simulink model "Solar_Plant_Harness"  (R2025b)
settings: Solver=VariableStepAuto  StartTime=0.0  StopTime=5  RelTol=1e-3
PostLoadFcn:
  | SolarPlantParam;
values from neighbouring files (symbols this model uses):
  Ts = 5E-5    (= 5e-05)    [BESSGFLParam.m]    (also in BESSGFMParam.m; WindFarmParam.m)
undefined symbols (not defined in the file or in its folder): ee_sli_rtmsupport, gcbh, PV, PVInverter, solar
libraries: nesl_utility x24, simulink x16, eeGeneralControl x12, ee_lib x11, slpidlib x6, eeTransforms x6, fl_lib x5, eeSinusoidalMeasurementV2 x2, eePwmGenerator x1, custom_lib x1
(part 1 of 3)
settings Model: SimulationMode=accelerator  Creator=skota  LastModifiedBy=skota

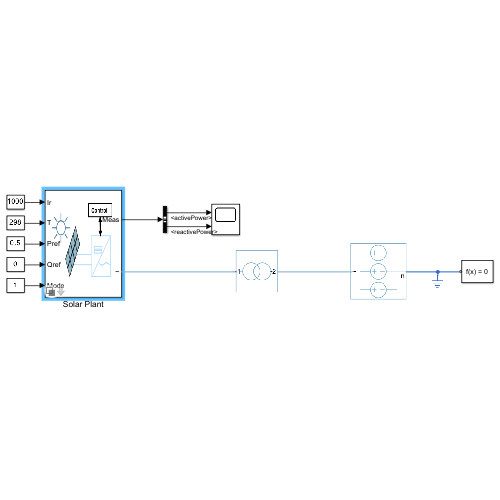
[thumbnail: Simulink's stored preview of the top-level diagram]
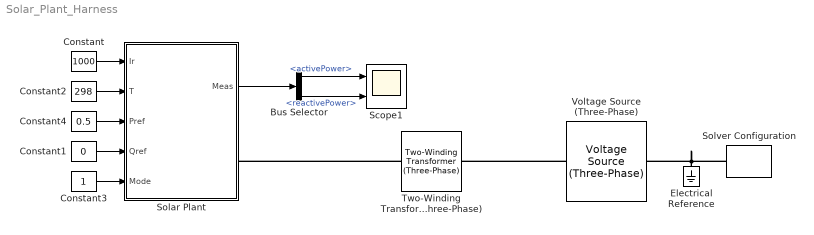
== system Solar_Plant_Harness ==
  Bus Selector : BusSelector  OutputSignals=activePower,reactivePower
  Constant : Constant  Value=1000  SampleTime=-1
  Constant1 : Constant  Value=0  SampleTime=-1
  Constant2 : Constant  Value=298  SampleTime=-1
  Constant3 : Constant  SampleTime=-1
  Constant4 : Constant  Value=0.5  SampleTime=-1
  Electrical Reference : fl_lib/Electrical/Electrical Elements/Electrical Reference
  Scope1 : Scope  NumInputPorts=2
      settings: ActiveDisplayYMinimum=-7.3875901679615126  ActiveDisplayYMaximum=4.8154652634596129  DataLoggingVariableName=ScopeData12
  Solar Plant : Subsystem  Variant=on  VariantControlMode=label  LabelModeActiveChoice=Detailed  mask(Solar){fidelity=Detailed, plantRating=PV.plantRating, Vac=PV.Vac, frequency=PV.frequency, iMaxPU=PVInverter.iMaxPU, efficiency=PV.converterEfficiency, baseVoltageDC=PV.baseVoltageDC, nParallel=536, nSeries=30, capacitance=PVInverter.capacitance, filterInductance=PVInverter.filterInductance, filterResistance=PVInverter.filterResistance, panelType=Poly-crystalline, panelRating=PV.panelRating, Isc=PV.Isc, Voc=PV.Voc, irradianceSTC=PV.irradianceSTC, temperatureSTC=PV.temperatureSTC, alpha=PV.alpha, beta=PV.beta, mode=Maximum power point tracking, converterFidelity=Average, fSw=PV.switchingFrequency}
      mask prompts: fidelity "Modeling Option"; plantRating "Solar Plant Rating (kW)"; Vac "Rated AC side voltage (phase-phase RMS) (V)"; frequency "Rated electrical frequency at AC side (Hz)"; iMaxPU "Maximum converter current (pu)"; efficiency "Converter Efficiency (%)"; baseVoltageDC "Voltage on DC side (V)"; nParallel "Number of panels in parallel"; nSeries "Number of panels in series"; capacitance "DC bus capacitance (F)"; filterInductance "Filter inductance (H)"; filterResistance "Filter series resistance (Ohm)"; panelType "Panel Type"; panelRating "Panel Rating (W)"; Isc "Short-circuit current (A)"; Voc "Open-circuit voltage (V)"; irradianceSTC "Irradiance at STC (W/m² )"; temperatureSTC "Temperature at STC (°K)"; alpha "Temperature co-efficient for current (A/°K)"; beta "Temperature co-efficient for voltage (V/°K)"; mode "Operating Mode"; converterFidelity "Converter Fidelity"; fSw "Switching Frequency (kHz)"
      mask help: This block models a Solar PV plant. The detailed variant models MPPT, voltage and current controllers. The simplified variant is based on Anderson's translational equations. Select simplified mode for faster simulation using fixed efficiency and rated power.
      settings: CopyFcn=set_param(gcbh,'LinkStatus','none');
      mask Help: web('SolarPlant.html')
      mask TypeOptions fidelity: Detailed | Simplified
      mask Callback fidelity: component.mask.fidelitySelection;
      mask TypeOptions nParallel: Detailed/PV Plant & Controller/PV Plant/nParallel
      mask TypeOptions nSeries: Detailed/PV Plant & Controller/PV Plant/nSeries
      mask TypeOptions panelType: Poly-crystalline | Mono-crystalline | Cadmium-Telluride | Others
      mask Callback panelType: component.mask.selectSolarPanelType;
      mask TypeOptions mode: Maximum power point tracking | Power reference
      mask Callback mode:
      | % choice = get_param(gcb,'mode');
      | % blockPath = [gcb,'/','Solar','/','Simplified','/','Solar_Plant'];
      | % blockHandle = get_param(blockPath, 'Handle');
      | % if strcmp(choice,'Maximum power point tracking')
      | %     set_param(blockPath,'modelling_option','ModellingOption.maximumPower');
      | % else
      | %     set_param(blockPath,'modelling_option','ModellingOption.powerReference');
      | % end
      mask TypeOptions converterFidelity: Detailed/PV Plant & Controller/PV Plant/converterFidelity
      mask Callback converterFidelity: component.mask.setSwitchingFrequency;
      mask TypeOptions fSw: Detailed/PV Plant & Controller/PV Plant/fSw
      mask DialogControl generalDetailed Prompt: General
      mask DialogControl cellDetailed Prompt: Solar Cell
      mask DialogControl partsCatalog Prompt: Click to choose from parts catalog
      mask DialogControl partsCatalog Callback: component.mask.openParamManager;
      mask DialogControl panelCalculation Prompt: Calculate number of panels
      mask DialogControl panelCalculation Callback: component.mask.setPanelNumber;
      mask DialogControl configureSolarCell Prompt: Edit Solar Cell Parameters
      mask DialogControl configureSolarCell Callback:
      | blockPath = [gcb,'/','Detailed','/','PV Plant & Controller','/','PV Plant','/','PV Array'];
      |     component.mask.openBlock(blockPath);
      mask DialogControl controllerDetailed Prompt: Solar PV Controller
      mask DialogControl configurePVController Prompt: Edit MPPT Controller
      mask DialogControl configurePVController Callback:
      | blockPath = [gcb,'/','Detailed','/','PV Plant & Controller','/','Controller','/','MPPT','/','Solar PV Controller'];
      |     component.mask.openBlock(blockPath);
      mask DialogControl configurePRefControl Prompt: Edit Power Reference Controller
      mask DialogControl configurePRefControl Callback:
      | blockPath = [gcb,'/','Detailed','/','PV Plant & Controller','/','Controller','/','Power Reference','/','Power Reference Controller'];
      |     component.mask.openBlock(blockPath);
      mask DialogControl cellSimplified Prompt: Solar Cell
      mask DialogControl converter Prompt: Converter
      mask DialogControl editConverter Prompt: Edit converter parameters
      mask DialogControl editConverter Callback:
      | converterFidelity = get_param(gcb,'converterFidelity');
      | blockPath = [gcb,'/','Detailed','/','PV Plant & Controller','/','PV Plant','/','Converter','/',converterFidelity,'/','Converter'];
      | component.mask.openBlock(blockPath);
      mask Display: image('solarPlant.png');
  Solver Configuration : nesl_utility/Solver Configuration  PhysicalDomain=network_engine_domain  SubClassName=solver  LeftPortType=input  RightPortType=generic  Tones=[]  Harmonics=[]  SimulateNoise=off  Profile=off  UseLocalSampling=off  EnableSwitchedLinearOptims=on  FrequencyDomain=off  UseCCode=off  RelTol=0.001  AbsTol=0.001  MinStep=1e-09  ToWorkspace=off  RevertToSquareIcSolve=off  NumHomotopyIterations=100  PhasorMode=off  PhasorModeNumHarmonics=1  ConsistencySolver=NEWTON_XTOL_AFTER_FTOL  IndexReductionMethod=DerivativeReplacement  DoDC=off  ResidualTolerance=1e-09  ConsistencyTolSource=GLOBAL  ConsistencyAbsTol=0.001  ConsistencyRelTol=0.001  ConsistencyTolFactor=0.001  UseLocalSolver=on  LocalSolverChoice=NE_BACKWARD_EULER_ADVANCER  ResolveIndetEquations=off  FunctionEvalNumThread=1  LocalSolverSampleTime=5e-5  DoFixedCost=on  MaxNonlinIter=1  MaxModeIter=2  ComputeImpulses=off  ImpulseIterations=2  LinearAlgebra=Sparse  LinearAlgebraNumThread=0  EquationFormulation=NE_TIME_EF  DelaysMemoryBudget=1024  AutomaticFiltering=off  FilteringTimeConstant=0.001  PartitionStorageMethod=AS_NEEDED  PartitionMemoryBudget=1024  PartitionMethod=ROBUST  MultibodyUseLocalSolver=off  MultibodyLocalSolverChoice=ODE1  MultibodyLocalSolverSampleTime=0.001
  Two-Winding Transformer (Three-Phase) : ee_lib/Passive/Transformers/Two-Winding Transformer (Three-Phase)  SRated=100e6 A*V  FRated=50 Hz  Winding1Connection=ee.enum.windingconnection.Yg  VRated1=690 V  Winding2Connection=ee.enum.windingconnection.Yg  VRated2=6600 V  CoreType=ee.enum.coretype.threelimb  pu_Rw1=0.01  pu_Rw2=0.01  leakage_reactance_option=ee.enum.transformer_leakage.include  pu_Xl1=0.05  pu_Xl2=0.05  magnetizing_resistance_option=ee.enum.transformer_magnetizingResistance.exclude  pu_Rm=500  magnetizing_reactance_option=ee.enum.transformer_magnetizingReactance.exclude  saturation_option=ee.enum.transformer_saturation.exclude  pu_Xm=500  current_data=[0, .002, 1, 2]  magnetic_flux_data=[0, 1.2, 1.5, 1.51]  pu_X0=0.5  i1_specify=off  i1_priority=None  i1=[0, 0, 0] A  i1_nominal_specify=off  i1_nominal_value=1  i1_nominal_unit=A  i2_specify=off  i2_priority=None  i2=[0, 0, 0] A  i2_nominal_specify=off  i2_nominal_value=1  i2_nominal_unit=A  phi_specify=off  phi_priority=None  phi=[0, 0, 0]  phi_nominal_specify=off  phi_nominal_value=1  phi_nominal_unit=1  power_dissipated_specify=off  power_dissipated_priority=None  power_dissipated=0 W  power_dissipated_nominal_specify=off  power_dissipated_nominal_value=1  power_dissipated_nominal_unit=W
      settings: InternalSimscapePortConfiguration="{\"Bottom\":[],\"Left\":[{\"id\":\"N1\",\"label\":\"~1\",\"type\":\"foundation.electrical.three_phase\"}],\"Right\":[{\"id\":\"N2\",\"label\":\"~2\",\"type\":\"foundation.electrical.three_phase\"}],\"Top\":[]}"
  Voltage Source (Three-Phase) : ee_lib/Sources/Voltage Source (Three-Phase)  vline_rms=6600 V  shift=0 deg  freq=50 Hz  impedance_option=0  SShortCircuit=1e6 A*V  XR=15  R=0.01 Ohm  L=3.97e-4 H  harmonic_option=0  harmonic_orders=[5, 7, 11, 13]  harmonic_ratios=[.1, .1, .1, .1]  G_parasitic=0 1/Ohm  I_specify=off  I_priority=None  I=[0, 0, 0] A  I_nominal_specify=off  I_nominal_value=1  I_nominal_unit=A
  wires:
  Constant1/1 -> Solar Plant/4(Qref)
  Constant2/1 -> Solar Plant/2(T)
  Constant3/1 -> Solar Plant/5(Mode)
  Constant4/1 -> Solar Plant/3(Pref)
  Constant/1 -> Solar Plant/1(Ir)
  Solar Plant/1(Meas) -> Bus Selector/1
  Bus Selector/1 -> Scope1/1  "<activePower>"
  Bus Selector/2 -> Scope1/2  "<reactivePower>"
  connections:
  Solver Configuration/RConn1 -- Electrical Reference/LConn1 -- Voltage Source (Three-Phase)/LConn1
  Two-Winding Transformer (Three-Phase)/LConn1 -- Solar Plant/RConn1
  Voltage Source (Three-Phase)/RConn1 -- Two-Winding Transformer (Three-Phase)/RConn1

== system Solar_Plant_Harness/Solar Plant ==
  Ir : Inport
  T : Inport  Port=2
  Pref : Inport  Port=3
  Qref : Inport  Port=4
  Mode : Inport  Port=5
  Detailed : Subsystem  VariantControl=Detailed
  Simplified : Subsystem  VariantControl=Simplified
  ~ : PMIOPort  Side=Right
  Meas : Outport

== system Solar_Plant_Harness/Solar Plant/Detailed ==
  Ir : Inport
  T : Inport  Port=2
  Pref : Inport  Port=3
  Qref : Inport  Port=4
  Mode : Inport  Port=5
  L Filter2 : ee_lib/Passive/RLC Assemblies/RLC (Three-Phase)  port_option=ee.enum.threePhasePort.composite  component_structure=ee.enum.rlc.structure.SeriesRL  R=filterResistance Ohm  L=filterInductance H  C=1e-6 F  R_parasitic=0 Ohm  G_parasitic=0 1/Ohm  IL_specify=on  IL_priority=None  IL=[0, 0, 0] A  IL_nominal_specify=off  IL_nominal_value=1  IL_nominal_unit=A  VC_specify=off  VC_priority=High  VC=[0, 0, 0] V  VC_nominal_specify=off  VC_nominal_value=1  VC_nominal_unit=V
      settings: InternalSimscapePortConfiguration="{\"Bottom\":[],\"Left\":[{\"id\":\"N1\",\"label\":\"~1\",\"type\":\"foundation.electrical.three_phase\"}],\"Right\":[{\"id\":\"N2\",\"label\":\"~2\",\"type\":\"foundation.electrical.three_phase\"}],\"Top\":[]}"
  Measurements : Subsystem
  PV Plant & Controller : Subsystem
  Terminator : Terminator
  ~ : PMIOPort  Side=Right
  Out Bus Element23 : Outport  PortName=Meas  Element=activePower
  Out Bus Element1 : Outport  PortName=Meas  Element=reactivePower
  Out Bus Element2 : Outport  PortName=Meas  Element=voltage
  Out Bus Element3 : Outport  PortName=Meas  Element=current
  wires:
  Measurements/2(Q) -> Out Bus Element1/1
  Measurements/4(I) -> Out Bus Element3/1, PV Plant & Controller/5(Iabc)
  Qref/1 -> PV Plant & Controller/3(Qref)
  Ir/1 -> PV Plant & Controller/1(Insolation)
  Measurements/3(V) -> Out Bus Element2/1, PV Plant & Controller/4(Vabc)
  Measurements/1(P) -> Out Bus Element23/1
  T/1 -> Terminator/1
  Pref/1 -> PV Plant & Controller/2(Pref)
  Mode/1 -> PV Plant & Controller/6(Mode)
  connections:
  L Filter2/RConn1 -- Measurements/LConn1
  L Filter2/LConn1 -- PV Plant & Controller/RConn1
  Measurements/RConn1 -- ~/RConn1

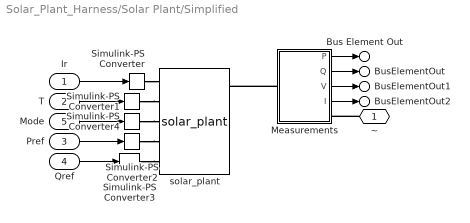
== system Solar_Plant_Harness/Solar Plant/Simplified ==
  Ir : Inport
  T : Inport  Port=2
  Pref : Inport  Port=3
  Qref : Inport  Port=4
  Mode : Inport  Port=5
  Measurements : Subsystem
  Simulink-PS Converter{,1..4} (5 alike) : nesl_utility/Simulink-PS Converter  PhysicalDomain=network_engine_domain  SubClassName=ps_input  LeftPortType=input  RightPortType=output  PseudoPeriodic=off  Frequencies=[]  NoiseDistribution=none  NoiseParameters=[]  Unit=1  AffineConversion=off  FilteringAndDerivatives=provide  SimscapeFilterOrder=1  InputFilterTimeConstant=0.001  UdotUserProvided=0
  solar_plant : custom_lib/solar_plant  port_option=ee.enum.threePhasePort.composite  FRated=frequency Hz  VRated=Vac V  PlantRating=plantRating kW  modelling_option=ModellingOption.powerReference  Vdc=2*Vac*sqrt(2/3) V  IMaxPU=iMaxPU  efficiency=efficiency  IrRef=irradianceSTC W/m^2  T=temperatureSTC K  PVTech=PanelTechnology.polycrystallinePanel  PanelRating=panelRating W  VocRef=Voc V  IscRef=Isc A  alpha=alpha 1/K  beta=beta 1/K  delta=0.111
      settings: InternalSimscapePortConfiguration="{\"Bottom\":[],\"Left\":[{\"id\":\"Ir\",\"label\":\"Ir\",\"type\":\"input\"},{\"id\":\"Tsim\",\"label\":\"T\",\"type\":\"input\"},{\"id\":\"Mode\",\"label\":\"Mode\",\"type\":\"input\"},{\"id\":\"Pref\",\"label\":\"Pref\",\"type\":\"input\"},{\"id\":\"Qref\",\"label\":\"Qref\",\"type\":\"input\"}],\"Right\":[{\"id\":\"N\",\"label\":\"~\",\"type\":\"foundation.electrical.three_phase\"},{\"id\":\"l\",\"label\":\"l\",\"type\":\"output\"},{\"id\":\"p\",\"label\":\"p\",\"type\":\"output\"}],\"Top\":[]}"
  ~ : PMIOPort  Side=Right
  Bus Element Out : Outport  PortName=Meas  Element=activePower
  BusElementOut : Outport  PortName=Meas  Element=reactivePower
  BusElementOut1 : Outport  PortName=Meas  Element=voltage
  BusElementOut2 : Outport  PortName=Meas  Element=current
  wires:
  Measurements/4(I) -> BusElementOut2/1
  Measurements/3(V) -> BusElementOut1/1
  Measurements/2(Q) -> BusElementOut/1
  Measurements/1(P) -> Bus Element Out/1
  Ir/1 -> Simulink-PS Converter/1
  T/1 -> Simulink-PS Converter1/1
  Pref/1 -> Simulink-PS Converter2/1
  Qref/1 -> Simulink-PS Converter3/1
  Mode/1 -> Simulink-PS Converter4/1
  connections:
  Simulink-PS Converter3/RConn1 -- solar_plant/LConn5
  Simulink-PS Converter4/RConn1 -- solar_plant/LConn3
  ~/RConn1 -- Measurements/RConn1
  Measurements/LConn1 -- solar_plant/RConn1
  Simulink-PS Converter/RConn1 -- solar_plant/LConn1
  Simulink-PS Converter1/RConn1 -- solar_plant/LConn2
  Simulink-PS Converter2/RConn1 -- solar_plant/LConn4

== system Solar_Plant_Harness/Solar Plant/Detailed/Measurements ==
  Current and Voltage Sensor (Three-Phase)5 : ee_lib/Sensors & Transducers/Current and Voltage Sensor (Three-Phase)  vMeasurementType=ee.enum.vmeasurement.lg  outputUnit=ee.enum.unit.pu  SRated=plantRating*1000 A*V  VRated=Vac V  I_specify=off  I_priority=None  I=[0, 0, 0] A  I_nominal_specify=off  I_nominal_value=1  I_nominal_unit=A  V_specify=off  V_priority=None  V=[0, 0, 0] V  V_nominal_specify=off  V_nominal_value=1  V_nominal_unit=V
      settings: InternalSimscapePortConfiguration="{\"Bottom\":[],\"Left\":[{\"id\":\"N1\",\"label\":\"~1\",\"type\":\"foundation.electrical.three_phase\"}],\"Right\":[{\"id\":\"V_output\",\"label\":\"V\",\"type\":\"output\"},{\"id\":\"I_output\",\"label\":\"I\",\"type\":\"output\"},{\"id\":\"N2\",\"label\":\"~2\",\"type\":\"foundation.electrical.three_phase\"}],\"Top\":[]}"
  Gain : Gain  Gain=1/(plantRating*1000)
  Gain1 : Gain  Gain=1/(plantRating*1000)
  Low-Pass Filter (Discrete or Continuous)1 : eeGeneralControl/Low-Pass Filter (Discrete or Continuous)  K=1  T=0.1  B=inf  A=-inf  init_option=Inherited from block input  x0=0  Ts=-1
  Low-Pass Filter (Discrete or Continuous)2 : eeGeneralControl/Low-Pass Filter (Discrete or Continuous)  K=1  T=0.1  B=inf  A=-inf  init_option=Inherited from block input  x0=0  Ts=-1
  PS-Simulink Converter{,1..3} (4 alike) : nesl_utility/PS-Simulink Converter  PhysicalDomain=network_engine_domain  SubClassName=ps_output  LeftPortType=input  RightPortType=output  PseudoPeriodic=off  Frequencies=[]  VectorFormat=inherit  Unit=inherit  AffineConversion=off
  Power Sensor (Three-Phase) : ee_lib/Sensors & Transducers/Power Sensor (Three-Phase)  load_type=ee.enum.passive.type_balanced.balanced  f0=60 Hz
      settings: InternalSimscapePortConfiguration="{\"Bottom\":[],\"Left\":[{\"id\":\"N1\",\"label\":\"~1\",\"type\":\"foundation.electrical.three_phase\"}],\"Right\":[{\"id\":\"N2\",\"label\":\"~2\",\"type\":\"foundation.electrical.three_phase\"}],\"Top\":[{\"id\":\"Pm\",\"label\":\"P\",\"type\":\"output\"},{\"id\":\"Qm\",\"label\":\"Q\",\"type\":\"output\"}]}"
  In : PMIOPort  Side=Left
  ~ : PMIOPort  Port=2  Side=Right
  P : Outport
  Q : Outport  Port=2
  V : Outport  Port=3
  I : Outport  Port=4
  wires:
  Gain1/1 -> Q/1
  Gain/1 -> P/1
  PS-Simulink Converter3/1 -> I/1
  PS-Simulink Converter2/1 -> V/1
  Low-Pass Filter (Discrete or Continuous)2/1 -> Gain1/1
  Low-Pass Filter (Discrete or Continuous)1/1 -> Gain/1
  PS-Simulink Converter1/1 -> Low-Pass Filter (Discrete or Continuous)2/1
  PS-Simulink Converter/1 -> Low-Pass Filter (Discrete or Continuous)1/1
  connections:
  PS-Simulink Converter3/LConn1 -- Current and Voltage Sensor (Three-Phase)5/RConn2
  Power Sensor (Three-Phase)/RConn1 -- Current and Voltage Sensor (Three-Phase)5/LConn1
  PS-Simulink Converter1/LConn1 -- Power Sensor (Three-Phase)/LConn3
  ~/RConn1 -- Current and Voltage Sensor (Three-Phase)5/RConn3
  In/RConn1 -- Power Sensor (Three-Phase)/LConn1
  PS-Simulink Converter/LConn1 -- Power Sensor (Three-Phase)/LConn2
  PS-Simulink Converter2/LConn1 -- Current and Voltage Sensor (Three-Phase)5/RConn1

== system Solar_Plant_Harness/Solar Plant/Detailed/PV Plant & Controller ==
  note: Controller
  note: Plant
  Insolation : Inport
  Pref : Inport  Port=2
  Qref : Inport  Port=3
  Vabc : Inport  Port=4
  Iabc : Inport  Port=5
  Mode : Inport  Port=6
  Controller : Subsystem
  Delay : Delay  DelayLength=1
  PV Plant : Subsystem  InitFcn=%solar.mask.restoreSolarLink(gcb);  mask(Solar Plant){capDC=capacitance, converterFidelity=Average, fSw=fSw, ratedVoltage=Vac, nSeries=nSeries, nParallel=nParallel}
      mask prompts: capDC "DC bus capacitance (F)"; converterFidelity "Converter Fidelity"; fSw "Switching Frequency (kHz)"; ratedVoltage "Rated voltage on AC side (V)"; nSeries "Number of panels in series"; nParallel "Number of panels in parallel"
      mask help: This block represents the physical interface between the solar panels and the power converter. It models the electrical and dynamic characteristics of the solar panels connected to a converter, while expecting an external control signal for operation
      settings: CopyFcn=set_param(gcbh,'LinkStatus','none');  PreSaveFcn=%solar.mask.restoreSolarLink(gcb);  CloseFcn=%solar.mask.restoreSolarLink(gcb);
      mask TypeOptions converterFidelity: Converter/converterFidelity
      mask Callback converterFidelity: component.mask.converterFidelityPlant;
      mask TypeOptions fSw: Converter/fSw
      mask DialogControl Container4 Prompt: General
      mask DialogControl editSolarCell Prompt: Edit Solar Cell Parameters
      mask DialogControl editSolarCell Callback:
      | blockPath = [gcb,'/','PV Array'];
      | component.mask.openBlock(blockPath);;
      mask DialogControl editConverter Prompt: Edit converter parameters
      mask DialogControl editConverter Callback:
      | converterFidelity = get_param(gcb,'converterFidelity');
      | blockPath = [gcb,'/','Converter','/',converterFidelity,'/','Converter'];
      | component.mask.openBlock(blockPath);
      mask Display: image('solar1.png');
  Scope1 : Scope
      settings: ActiveDisplayYMinimum=-2.35685  ActiveDisplayYMaximum=2.29234  DataLoggingVariableName=ScopeData4
  Sensor Dynamics : Subsystem
  Simulink-PS Converter : nesl_utility/Simulink-PS Converter  PhysicalDomain=network_engine_domain  SubClassName=ps_input  LeftPortType=input  RightPortType=output  PseudoPeriodic=off  Frequencies=[]  NoiseDistribution=none  NoiseParameters=[]  Unit=1  AffineConversion=off  FilteringAndDerivatives=provide  SimscapeFilterOrder=1  InputFilterTimeConstant=0.001  UdotUserProvided=0
  abc : PMIOPort  Side=Right
  wires:
  PV Plant/2(V) -> Sensor Dynamics/2(Vin)
  PV Plant/1(I) -> Sensor Dynamics/1(Iin)
  Delay/1 -> PV Plant/1(mabc)
  Insolation/1 -> Simulink-PS Converter/1
  Controller/1(vabcRef (pu)) -> Scope1/1, Delay/1
  Sensor Dynamics/2(V) -> Controller/3(vdc (V))
  Sensor Dynamics/1(I) -> Controller/2(ipv (A))
  Qref/1 -> Controller/1(Qref)
  Pref/1 -> Controller/6(Pref)
  Vabc/1 -> Controller/4(Vabc)
  Iabc/1 -> Controller/5(Iabc)
  Mode/1 -> Controller/7(Mode)
  connections:
  abc/RConn1 -- PV Plant/RConn1
  PV Plant/LConn1 -- Simulink-PS Converter/RConn1

== system Solar_Plant_Harness/Solar Plant/Simplified/Measurements ==
  Current and Voltage Sensor (Three-Phase)5 : ee_lib/Sensors & Transducers/Current and Voltage Sensor (Three-Phase)  vMeasurementType=ee.enum.vmeasurement.lg  outputUnit=ee.enum.unit.pu  SRated=plantRating*1000 A*V  VRated=Vac V  I_specify=off  I_priority=None  I=[0, 0, 0] A  I_nominal_specify=off  I_nominal_value=1  I_nominal_unit=A  V_specify=off  V_priority=None  V=[0, 0, 0] V  V_nominal_specify=off  V_nominal_value=1  V_nominal_unit=V
      settings: InternalSimscapePortConfiguration="{\"Bottom\":[],\"Left\":[{\"id\":\"N1\",\"label\":\"~1\",\"type\":\"foundation.electrical.three_phase\"}],\"Right\":[{\"id\":\"V_output\",\"label\":\"V\",\"type\":\"output\"},{\"id\":\"I_output\",\"label\":\"I\",\"type\":\"output\"},{\"id\":\"N2\",\"label\":\"~2\",\"type\":\"foundation.electrical.three_phase\"}],\"Top\":[]}"
  Gain : Gain  Gain=1/(plantRating*1000)
  Gain1 : Gain  Gain=1/(plantRating*1000)
  Low-Pass Filter (Discrete or Continuous)1 : eeGeneralControl/Low-Pass Filter (Discrete or Continuous)  K=1  T=0.1  B=inf  A=-inf  init_option=Inherited from block input  x0=0  Ts=-1
  Low-Pass Filter (Discrete or Continuous)2 : eeGeneralControl/Low-Pass Filter (Discrete or Continuous)  K=1  T=0.1  B=inf  A=-inf  init_option=Inherited from block input  x0=0  Ts=-1
  PS-Simulink Converter{,1..3} (4 alike) : nesl_utility/PS-Simulink Converter  PhysicalDomain=network_engine_domain  SubClassName=ps_output  LeftPortType=input  RightPortType=output  PseudoPeriodic=off  Frequencies=[]  VectorFormat=inherit  Unit=inherit  AffineConversion=off
  Power Sensor (Three-Phase) : ee_lib/Sensors & Transducers/Power Sensor (Three-Phase)  load_type=ee.enum.passive.type_balanced.balanced  f0=60 Hz
      settings: InternalSimscapePortConfiguration="{\"Bottom\":[],\"Left\":[{\"id\":\"N1\",\"label\":\"~1\",\"type\":\"foundation.electrical.three_phase\"}],\"Right\":[{\"id\":\"N2\",\"label\":\"~2\",\"type\":\"foundation.electrical.three_phase\"}],\"Top\":[{\"id\":\"Pm\",\"label\":\"P\",\"type\":\"output\"},{\"id\":\"Qm\",\"label\":\"Q\",\"type\":\"output\"}]}"
  In : PMIOPort  Side=Left
  ~ : PMIOPort  Port=2  Side=Right
  P : Outport
  Q : Outport  Port=2
  V : Outport  Port=3
  I : Outport  Port=4
  wires:
  Gain1/1 -> Q/1
  Gain/1 -> P/1
  PS-Simulink Converter3/1 -> I/1
  PS-Simulink Converter2/1 -> V/1
  Low-Pass Filter (Discrete or Continuous)2/1 -> Gain1/1
  Low-Pass Filter (Discrete or Continuous)1/1 -> Gain/1
  PS-Simulink Converter1/1 -> Low-Pass Filter (Discrete or Continuous)2/1
  PS-Simulink Converter/1 -> Low-Pass Filter (Discrete or Continuous)1/1
  connections:
  PS-Simulink Converter3/LConn1 -- Current and Voltage Sensor (Three-Phase)5/RConn2
  Power Sensor (Three-Phase)/RConn1 -- Current and Voltage Sensor (Three-Phase)5/LConn1
  PS-Simulink Converter1/LConn1 -- Power Sensor (Three-Phase)/LConn3
  ~/RConn1 -- Current and Voltage Sensor (Three-Phase)5/RConn3
  In/RConn1 -- Power Sensor (Three-Phase)/LConn1
  PS-Simulink Converter/LConn1 -- Power Sensor (Three-Phase)/LConn2
  PS-Simulink Converter2/LConn1 -- Current and Voltage Sensor (Three-Phase)5/RConn1

== system Solar_Plant_Harness/Solar Plant/Detailed/PV Plant & Controller/Controller ==
  Qref : Inport
  ipv (A) : Inport  Port=2
  vdc (V) : Inport  Port=3
  Vabc : Inport  Port=4
  Iabc : Inport  Port=5
  Pref : Inport  Port=6
  Mode : Inport  Port=7
  If : If
  MPPT : Subsystem  TreatAsAtomicUnit=on
  Merge : Merge
  Power Reference : Subsystem  TreatAsAtomicUnit=on
  vabcRef (pu) : Outport
  wires:
  ipv (A)/1 -> MPPT/2(ipv (A))
  vdc (V)/1 -> MPPT/3(vdc (V))
  Qref/1 -> MPPT/1(Qref), Power Reference/4(QRef)
  Iabc/1 -> Power Reference/1(Iabc), MPPT/5(Iabc)
  Pref/1 -> Power Reference/3(PRef)
  Vabc/1 -> Power Reference/2(Vabc), MPPT/4(Vabc)
  If/1 -> MPPT/Action
  If/2 -> Power Reference/Action
  MPPT/1(mabc) -> Merge/1
  Power Reference/1(mabc) -> Merge/2
  Merge/1 -> vabcRef (pu)/1
  Mode/1 -> If/1

== system Solar_Plant_Harness/Solar Plant/Detailed/PV Plant & Controller/PV Plant ==
  mabc : Inport
  Converter : Subsystem  InitFcn=%solar.mask.restoreConverterLink(gcb);  Variant=on  VariantControlMode=label  LabelModeActiveChoice=Average  mask{converterFidelity=Average, fSw=fSw}
      mask prompts: converterFidelity "Converter Fidelity"; fSw "Switching Frequency (kHz)"
      settings: PreSaveFcn=%solar.mask.restoreConverterLink  CloseFcn=%solar.mask.restoreConverterLink
      mask TypeOptions converterFidelity: Average | Switching
      mask Callback converterFidelity: component.mask.converterFidelity(gcb);
      mask DialogControl editSwitch Prompt: Edit converter parameters
      mask DialogControl editSwitch Callback:
      | converterFidelity = get_param(gcb,'converterFidelity');
      | blockPath = [gcb,'/',converterFidelity,'/','Converter'];
      | component.mask.openBlock(blockPath);
  Current Sensor : fl_lib/Electrical/Electrical Sensors/Current Sensor
  DC- Capacitor : fl_lib/Electrical/Electrical Elements/Capacitor  c=capDC F  r=1e-6 Ohm  g=0 1/Ohm  i_specify=off  i_priority=None  i=0 A  i_nominal_specify=off  i_nominal_value=1  i_nominal_unit=A  v_specify=off  v_priority=None  v=6560*.5 V  v_nominal_specify=off  v_nominal_value=1  v_nominal_unit=V  vc_specify=on  vc_priority=None  vc=ceil(Vac*sqrt(2)*1.2) V  vc_nominal_specify=off  vc_nominal_value=1  vc_nominal_unit=V
  ERef1 : fl_lib/Electrical/Electrical Elements/Electrical Reference
  PS-Simulink Converter : nesl_utility/PS-Simulink Converter  PhysicalDomain=network_engine_domain  SubClassName=ps_output  LeftPortType=input  RightPortType=output  PseudoPeriodic=off  Frequencies=[]  VectorFormat=inherit  Unit=inherit  AffineConversion=off
  PS-Simulink Converter1 : nesl_utility/PS-Simulink Converter  PhysicalDomain=network_engine_domain  SubClassName=ps_output  LeftPortType=input  RightPortType=output  PseudoPeriodic=off  Frequencies=[]  VectorFormat=inherit  Unit=inherit  AffineConversion=off
  PV Array : ee_lib/Sources/Solar Cell  PartSpecification="{\"CollectionId\":\"SimscapeElectrical\",\"DatasetId\":\"Tata_Power_Solar|TP300|simscape.electrical.solarCell\",\"DisplayName\":\"Tata_Power_Solar:TP300\"}"  prm=ee.enum.sources.solar_cell_prm.fiveParameter  Isc=8.71 % Datasheet derived A  Voc=0.62223 % Datasheet derived V  Is=1.08146075786774e-06 % Datasheet derived A  Is2=5.42602984007438e-09 % Datasheet derived A  Iph=8.71000410148422 % Datasheet derived A  Ir0=1000 % Datasheet derived W/m^2  ec=1.52301308864556 % Datasheet derived  N2=1.87068753668451 % Datasheet derived  Rs=0.000339119125335165 % Datasheet derived Ohm  Rp=655.536158839936 % Datasheet derived Ohm  N_series=72*nSeries% Datasheet derived  N_parallel=1*nParallel % Datasheet derived  TIPH1=0.000579985599628516 % Datasheet derived 1/K  EG=1.12 % Datasheet derived eV  TXIS1=3.78147935095899 % Datasheet derived  TXIS2=12.1162776751811 % Datasheet derived  TRS1=0.141899818875295 % Datasheet derived  TRP1=0 % Parameter not set  Tmeas=25 % Datasheet derived degC  TFIXED=25 % Datasheet derived degC  thermal_mass=100 % Parameter not set J/K  initial_temperature=25 degC
      settings: AttributesFormatString=Tata_Power_Solar:TP300
  Voltage Sensor : fl_lib/Electrical/Electrical Sensors/Voltage Sensor
  ABC : PMIOPort  Side=Right
  Ir : PMIOPort  Port=2  Side=Left
  I : Outport
  V : Outport  Port=2
  wires:
  PS-Simulink Converter/1 -> I/1
  PS-Simulink Converter1/1 -> V/1
  mabc/1 -> Converter/1(mabc)
  connections:
  PV Array/LConn2 -- Current Sensor/LConn1
  ABC/RConn1 -- Converter/RConn1
  Ir/RConn1 -- PV Array/LConn1
  PS-Simulink Converter/LConn1 -- Current Sensor/RConn1
  PS-Simulink Converter1/LConn1 -- Voltage Sensor/RConn1
  DC- Capacitor/LConn1 -- Converter/LConn1 -- Current Sensor/RConn2 -- Voltage Sensor/LConn1
  DC- Capacitor/RConn1 -- Converter/LConn2 -- ERef1/LConn1 -- PV Array/RConn1 -- Voltage Sensor/RConn2

== system Solar_Plant_Harness/Solar Plant/Detailed/PV Plant & Controller/Sensor Dynamics ==
  Iin : Inport
  Vin : Inport  Port=2
  Current Measurement : Subsystem
  Product : Product
  Scope : Scope
      settings: ActiveDisplayYMinimum=-1.17977100562E+6  ActiveDisplayYMaximum=5.50264896669E+6  DataLoggingVariableName=ScopeData5
  Voltage Measurement : Subsystem
  I : Outport
  V : Outport  Port=2
  wires:
  Current Measurement/1(V) -> Product/2, I/1
  Iin/1 -> Current Measurement/1(u)
  Vin/1 -> Voltage Measurement/1(u)
  Voltage Measurement/1(I) -> Product/1, V/1
  Product/1 -> Scope/1

== system Solar_Plant_Harness/Solar Plant/Detailed/PV Plant & Controller/Controller/MPPT ==
  Qref : Inport
  ipv (A) : Inport  Port=2
  vdc (V) : Inport  Port=3
  Vabc : Inport  Port=4
  Iabc : Inport  Port=5
  Action Port : ActionPort  ActionPortLabel=if(u1 > 0)
  Solar PV Controller : Subsystem  LoadFcn=ee_sli_rtmsupport( 'loadfcn', gcbh );  mask(Solar PV Controller (Three-Phase)){L=filterInductance, frequency=frequency, iMax=iMaxPU, zBase=Vac^2/(plantRating*1000), mVAbase=plantRating*1000, VdcBase=baseVoltageDC, sampleTime=-1, Choice=Perturb and observe (P&O), Vdc=1100, delV=3, tSettling=1e-3, Kppll=1e-4, Kipll=0.02, initialPhase=0, Kpv=PV.controllerKpv, Kiv=PV.controllerKiv, Kdv=0, Kpicd=PV.controllerKpIc, Kiicd=PV.controllerKiIc, Kdicd=0, Kpicq=PV.controllerKpIc, Kiicq=PV.controllerKiIc, Kdicq=0}
      mask prompts: L "physmod:ee:library:comments:control:eeRenewablesControl:ACFilterInductanceH_MP"; frequency "physmod:ee:library:comments:control:eeRenewablesControl:SystemFrequencyHz_MP"; iMax "physmod:ee:library:comments:control:eeRenewablesControl:InverterCurrentLimitpu_MP"; zBase "physmod:ee:library:comments:control:eeRenewablesControl:BaseImpedanceACSideOhm_MP"; mVAbase "physmod:ee:library:comments:control:eeRenewablesControl:BaseMVA_MP"; VdcBase "physmod:ee:library:comments:control:eeRenewablesControl:DCBusBaseVoltageV_MP"; sampleTime "physmod:ee:library:comments:control:eeRenewablesControl:SampleTime1ForInherited_MP"; Choice "physmod:ee:library:comments:control:eeRenewablesControl:Algorithm_MP"; Vdc "physmod:ee:library:comments:control:eeRenewablesControl:InitialVoltageForMPPTV_MP"; delV "physmod:ee:library:comments:control:eeRenewablesControl:VoltageStepOfMPPTV_MP"; tSettling "physmod:ee:library:comments:control:eeRenewablesControl:SettlingTimeOfMPPTs_MP"; Kppll "physmod:ee:library:comments:control:eeRenewablesControl:ProportionalGain_MP"; Kipll "physmod:ee:library:comments:control:eeRenewablesControl:IntegralGain_MP"; initialPhase "physmod:ee:library:comments:control:eeRenewablesControl:InitialPhaseAngle_MP"; Kpv "physmod:ee:library:comments:control:eeRenewablesControl:ProportionalGain_MP"; Kiv "physmod:ee:library:comments:control:eeRenewablesControl:IntegralGain_MP"; Kdv "physmod:ee:library:comments:control:eeRenewablesControl:DerivativeGain_MP"; Kpicd "physmod:ee:library:comments:control:eeRenewablesControl:DaxisProportionalGain_MP"; Kiicd "physmod:ee:library:comments:control:eeRenewablesControl:DaxisIntegralGain_MP"; Kdicd "physmod:ee:library:comments:control:eeRenewablesControl:DaxisDerivativeGain_MP"; Kpicq "physmod:ee:library:comments:control:eeRenewablesControl:QaxisProportionalGain_MP"; Kiicq "physmod:ee:library:comments:control:eeRenewablesControl:QaxisIntegralGain_MP"; Kdicq "physmod:ee:library:comments:control:eeRenewablesControl:QaxisDerivativeGain_MP"
      mask help: physmod:ee:library:comments:control:eeRenewablesControl:PVGridFollowingController_MD
      mask init:
      | timeDomain = ee.mask.getSampleTimeDomain(sampleTime,gcb);
      | if sampleTime < 0 && sampleTime ~= -1            
      |     error(message('physmod:ee:library:MinusOneZeroOrPositive',getString(message('physmod:ee:library:comments:control:eeRenewablesControl:SampleTime1ForInherited_MP'))));            
      | end
      | if L <= 0            
      |     error(message('physmod:simscape:compiler:patterns:checks:GreaterThanZero',getString(message('physmod:ee:library:comments:control:eeRenewablesControl:ACFilterInductanceH_MP'))));            
      | end
      | if VdcBase <= 0            
      |     error(message('physmod:simscape:compiler:patterns:checks:GreaterThanZero',getString(message('physmod:ee:library:comments:control:eeRenewablesControl:DCBusBaseVoltageV_MP'))));            
      | end
      | if delV <= 0            
      |     error(message('physmod:simscape:compiler:patterns:checks:GreaterThanZero',getString(message('physmod:ee:library:comments:control:eeRenewablesControl:VoltageStepOfMPPTV_MP'))));            
      | end
      | if tSettling <= 0            
      |     error(message('physmod:simscape:compiler:patterns:checks:GreaterThanZero',getString(message('physmod:ee:library:comments:control:eeRenewablesControl:SettlingTimeOfMPPTs_MP'))));            
      | end
      | if zBase <= 0            
      |     error(message('physmod:simscape:compiler:patterns:checks:GreaterThanZero',getString(message('physmod:ee:library:comments:control:eeRenewablesControl:BaseImpedanceACSideOhm_MP'))));            
      | end
      | if iMax <= 0            
      |     error(message('physmod:simscape:compiler:patterns:checks:GreaterThanZero',getString(message('physmod:ee:library:comments:control:eeRenewablesControl:InverterCurrentLimitpu_MP'))));            
      | end
      | if frequency <= 0            
      |     error(message('physmod:simscape:compiler:patterns:checks:GreaterThanZero',getString(message('physmod:ee:library:comments:control:eeRenewablesControl:SystemFrequencyHz_MP'))));            
      | end
      settings: CopyFcn=ee_sli_rtmsupport( 'copyfcn', gcbh );  DeleteFcn=ee_sli_rtmsupport( 'deletefcn', gcbh );  ModelCloseFcn=ee_sli_rtmsupport( 'modelclosefcn', gcbh );  PostSaveFcn=ee_sli_rtmsupport( 'postsavefcn', gcbh );  PreCopyFcn=ee_sli_rtmsupport( 'precopyfcn', gcbh );  OpenFcn=ee_sli_rtmsupport( 'openfcn', gcbh );  CloseFcn=ee_sli_rtmsupport( 'closefcn', gcbh );  PreDeleteFcn=ee_sli_rtmsupport( 'predeletefcn', gcbh );
      mask Help: web(nesl_help(gcbh))
      mask TypeOptions sampleTime: Current_controller/SystemSampleTime | DC voltage controller & current reference/SystemSampleTime
      mask TypeOptions Choice: Variant Subsystem/LabelModeActiveChoice
      mask DialogControl Container4 Prompt: physmod:ee:library:comments:control:eeRenewablesControl:General_Tab
      mask DialogControl L Prompt: AC filter inductance (H)
      mask DialogControl frequency Prompt: System frequency (Hz)
      mask DialogControl iMax Prompt: Inverter current limit (pu)
      mask DialogControl zBase Prompt: Base impedance on AC side (Ohm)
      mask DialogControl mVAbase Prompt: Base power on AC side (V*A)
      mask DialogControl VdcBase Prompt: DC bus base voltage (V)
      mask DialogControl sampleTime Prompt: Sample time (-1 for inherited)
      mask DialogControl Container5 Prompt: physmod:ee:library:comments:control:eeRenewablesControl:MPPT_Tab
      mask DialogControl Choice Prompt: Algorithm
      mask DialogControl Vdc Prompt: Initial voltage for MPPT (V)
      mask DialogControl delV Prompt: Voltage step of MPPT (V)
      mask DialogControl tSettling Prompt: Settling time of MPPT (s)
      mask DialogControl Container6 Prompt: physmod:ee:library:comments:control:eeRenewablesControl:PLL_Tab
      mask DialogControl Kppll Prompt: Proportional gain
      mask DialogControl Kipll Prompt: Integral gain
      mask DialogControl initialPhase Prompt: Initial phase angle (deg)
      mask DialogControl Container7 Prompt: physmod:ee:library:comments:control:eeRenewablesControl:VoltageController_Tab
      mask DialogControl Kpv Prompt: Proportional gain
      mask DialogControl Kiv Prompt: Integral gain
      mask DialogControl Kdv Prompt: Derivative gain
      mask DialogControl Container8 Prompt: physmod:ee:library:comments:control:eeRenewablesControl:CurrentController_Tab
      mask DialogControl Kpicd Prompt: D-axis proportional gain
      mask DialogControl Kiicd Prompt: D-axis integral gain
      mask DialogControl Kdicd Prompt: D-axis derivative gain
      mask DialogControl Kpicq Prompt: Q-axis proportional gain
      mask DialogControl Kiicq Prompt: Q-axis integral gain
      mask DialogControl Kdicq Prompt: Q-axis derivative gain
      mask Display: ee.mask.drawPVcontroller;
  mabc : Outport
  wires:
  ipv (A)/1 -> Solar PV Controller/2(ipv (A))
  Iabc/1 -> Solar PV Controller/5(iabc (pu))
  Vabc/1 -> Solar PV Controller/4(vabc (pu))
  vdc (V)/1 -> Solar PV Controller/3(vdc (V))
  Qref/1 -> Solar PV Controller/1(Qref (pu))
  Solar PV Controller/1(vabcRef (pu)) -> mabc/1

== system Solar_Plant_Harness/Solar Plant/Detailed/PV Plant & Controller/Controller/Power Reference ==
  Iabc : Inport
  Vabc : Inport  Port=2
  PRef : Inport  Port=3
  QRef : Inport  Port=4
  Action Port : ActionPort  ActionPortLabel=else
  Power Reference Controller : Subsystem  mask(Power Reference Controller){frequency=frequency, P=Real power, MVA=plantRating*1000, zbase=Vac^2/plantRating, L=filterInductance, Imax=iMaxPU, Td=1e-3, Kpic=1.5, Kiic=10, Kd=0, kpPLL=40, kiPLL=1000, kdPLL=0}
      mask prompts: frequency "Frequency (Hz)"; P "Priority mode"; MVA "Base Power (V*A)"; zbase "Base Impedance (Ohm)"; L "Filter Inductance (H)"; Imax "Inverter current limit (pu)"; Td "Sensor time delay (s)"; Kpic "Proportional gain"; Kiic "Integral gain"; Kd "Derevative gain"; kpPLL "Proportional gain"; kiPLL "Integral gain"; kdPLL "Derevative gain"
      mask help: This block receives active and reactive power references for the converter based on system requirements or higher-level control commands. It ensures that the converter operates according to desired power setpoints, supporting grid services such as frequency regulation, voltage support, and power dispatch
      settings: CopyFcn=set_param(gcbh,'LinkStatus','none');
      mask TypeOptions P: Real power  | Reactive power
      mask DialogControl Container4 Prompt: General
      mask DialogControl Container5 Prompt: Current Controller
      mask DialogControl Container5_copy Prompt: PLL
  mabc : Outport
  wires:
  QRef/1 -> Power Reference Controller/4(Qref)
  PRef/1 -> Power Reference Controller/3(Pref)
  Power Reference Controller/1(mabc) -> mabc/1
  Vabc/1 -> Power Reference Controller/2(Vabc)
  Iabc/1 -> Power Reference Controller/1(Iabc)

== system Solar_Plant_Harness/Solar Plant/Detailed/PV Plant & Controller/PV Plant/Converter ==
  mabc : Inport
  Average : Subsystem  VariantControl=Average
  Switching : Subsystem  VariantControl=Switching
  + : PMIOPort  Side=Left
  - : PMIOPort  Port=2  Side=Left
  ~ : PMIOPort  Port=3  Side=Right

== system Solar_Plant_Harness/Solar Plant/Detailed/PV Plant & Controller/Sensor Dynamics/Current Measurement ==
  u : Inport
  Lead-Lag (Discrete or Continuous) : eeGeneralControl/Lead-Lag (Discrete or Continuous)  T1=0  T2=PV.controllerTSensor  B=inf  A=-inf  init_option=Inherited from block input  x0=0  Ts=Ts
  V : Outport
  wires:
  u/1 -> Lead-Lag (Discrete or Continuous)/1
  Lead-Lag (Discrete or Continuous)/1 -> V/1

== system Solar_Plant_Harness/Solar Plant/Detailed/PV Plant & Controller/Sensor Dynamics/Voltage Measurement ==
  u : Inport
  Lead-Lag (Discrete or Continuous) : eeGeneralControl/Lead-Lag (Discrete or Continuous)  T1=0  T2=PV.controllerTSensor  B=inf  A=-inf  init_option=Inherited from block input  x0=0  Ts=Ts
  I : Outport
  wires:
  u/1 -> Lead-Lag (Discrete or Continuous)/1
  Lead-Lag (Discrete or Continuous)/1 -> I/1

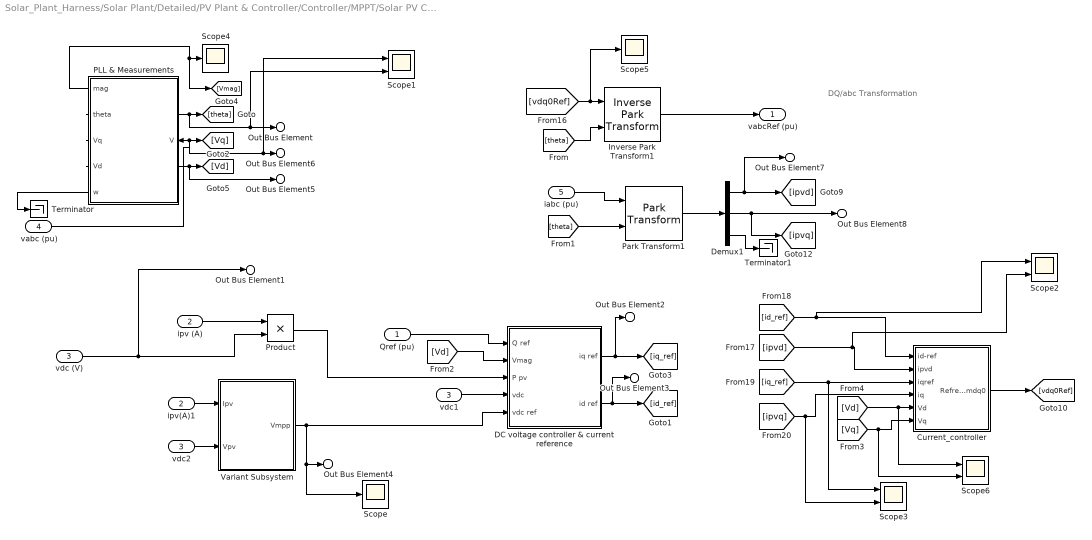
== system Solar_Plant_Harness/Solar Plant/Detailed/PV Plant & Controller/Controller/MPPT/Solar PV Controller ==
  note: DQ/abc Transformation
  Qref (pu) : Inport
  ipv (A) : Inport  Port=2
  vdc (V) : Inport  Port=3
  vabc (pu) : Inport  Port=4
  iabc (pu) : Inport  Port=5
  Current_controller : Subsystem  SystemSampleTime=sampleTime
  DC voltage controller & current reference : Subsystem  SystemSampleTime=sampleTime
  Demux1 : Demux  Outputs=3
  Inverse Park Transform1 : eeTransforms/Inverse Park Transform  AxisAlignment=Q-axis  PowerInvariant=off
  PLL & Measurements : Subsystem
  Park Transform1 : eeTransforms/Park Transform  AxisAlignment=Q-axis  PowerInvariant=off
  Product : Product
  Scope : Scope
      settings: ActiveDisplayYMinimum=719.47133  ActiveDisplayYMaximum=1441.72759  DataLoggingVariableName=ScopeData5
  Scope{1..3,6} (4 alike) : Scope  NumInputPorts=2
      Scope1 settings: ActiveDisplayYMinimum=-0.55297  ActiveDisplayYMaximum=0.65726  DataLoggingVariableName=ScopeData6
      Scope2 settings: ActiveDisplayYMinimum=0.74203  ActiveDisplayYMaximum=1.09578
      Scope3 settings: ActiveDisplayYMinimum=-1  ActiveDisplayYMaximum=1
      Scope6 settings: ActiveDisplayYMinimum=0.97205  ActiveDisplayYMaximum=1.00522  DataLoggingVariableName=ScopeData6
  Scope4 : Scope
      settings: ActiveDisplayYMinimum=-0.12504  ActiveDisplayYMaximum=1.12534
  Scope5 : Scope
      settings: ActiveDisplayYMinimum=-0.12621  ActiveDisplayYMaximum=1.13592
  Terminator : Terminator
  Terminator1 : Terminator
  Variant Subsystem : Subsystem  Variant=on  VariantControlMode=label  LabelModeActiveChoice=Perturb and observe (P&O)
  ipv(A)1 : InportShadow  Port=2
  vdc1 : InportShadow  Port=3
  vdc2 : InportShadow  Port=3
  vabcRef (pu) : Outport
  Out Bus Element : Outport  Port=2  PortName=visualization  Element=theta [rad]
  Out Bus Element1 : Outport  Port=2  PortName=visualization  Element=vdc [Volts]
  Out Bus Element2 : Outport  Port=2  PortName=visualization  Element=iq ref [pu]
  Out Bus Element3 : Outport  Port=2  PortName=visualization  Element=id ref [pu]
  Out Bus Element4 : Outport  Port=2  PortName=visualization  Element=vdc ref [Volts]
  Out Bus Element5 : Outport  Port=2  PortName=visualization  Element=Vd [pu]
  Out Bus Element6 : Outport  Port=2  PortName=visualization  Element=Vq [pu]
  Out Bus Element7 : Outport  Port=2  PortName=visualization  Element=id [pu]
  Out Bus Element8 : Outport  Port=2  PortName=visualization  Element=iq [pu]
  wires:
  PLL & Measurements/2(theta) -> [theta], Scope1/2, Out Bus Element/1
  ipv(A)1/1 -> Variant Subsystem/1(Ipv)
  vdc2/1 -> Variant Subsystem/2(Vpv)
  ipv (A)/1 -> Product/1
  PLL & Measurements/5(w) -> Terminator/1
  Variant Subsystem/1(Vmpp) -> DC voltage controller & current reference/5(vdc ref), Scope/1, Out Bus Element4/1
  vdc1/1 -> DC voltage controller & current reference/4(vdc)
  vabc (pu)/1 -> PLL & Measurements/1(V)
  PLL & Measurements/4(Vd) -> [Vd], Out Bus Element5/1
  PLL & Measurements/1(mag) -> Scope4/1, [Vmag]
  PLL & Measurements/3(Vq) -> [Vq], Scope1/1, Out Bus Element6/1
  Product/1 -> DC voltage controller & current reference/3(P pv)
  vdc (V)/1 -> Product/2, Out Bus Element1/1
  Qref (pu)/1 -> DC voltage controller & current reference/1(Q ref)
  DC voltage controller & current reference/2(id ref) -> [id_ref], Out Bus Element3/1
  DC voltage controller & current reference/1(iq ref) -> [iq_ref], Out Bus Element2/1
  [Vd] -> DC voltage controller & current reference/2(Vmag)
  iabc (pu)/1 -> Park Transform1/1
  [ipvd] -> Scope2/2, Current_controller/2(ipvd)
  [theta] -> Inverse Park Transform1/2
  [theta] -> Park Transform1/2
  [ipvq] -> Scope3/2, Current_controller/4(iq)
  [iq_ref] -> Scope3/1, Current_controller/3(iqref)
  [Vd] -> Scope6/1, Current_controller/5(Vd)
  [id_ref] -> Scope2/1, Current_controller/1(id-ref)
  Park Transform1/1 -> Demux1/1
  [vdq0Ref] -> Scope5/1, Inverse Park Transform1/1
  Demux1/3 -> Terminator1/1
  Demux1/1 -> [ipvd], Out Bus Element7/1
  Inverse Park Transform1/1 -> vabcRef (pu)/1
  Demux1/2 -> [ipvq], Out Bus Element8/1
  Current_controller/1(Refrence_mdq0) -> [vdq0Ref]
  [Vq] -> Scope6/2, Current_controller/6(Vq)

== system Solar_Plant_Harness/Solar Plant/Detailed/PV Plant & Controller/Controller/Power Reference/Power Reference Controller ==
  Iabc : Inport
  Vabc : Inport  Port=2
  Pref : Inport  Port=3
  Qref : Inport  Port=4
  Constant : Constant  Value=10
  PLL & Measurements : Subsystem
      mask Display: image('$imagefile'); % Use "Edit Image" on toolstrip to change.
  Power Reference Controller : Subsystem  mask{mp=0, mv=0, P=Real power, MVA=MVA, zbase=Vac^2/(MVA), L=L, Imax=Imax, Td=1e-3, Kpic=Kpic, Kiic=Kiic, Kd=0}
      mask prompts: mp "Real power droop cofficient"; mv "Reactive power droop cofficient"; P "Priority mode"; MVA "Base Power (V*A)"; zbase "Base Impedance (Ohm)"; L "Filter Inductance (H)"; Imax "Inverter current limit (pu)"; Td "Sensor time delay (s)"; Kpic "Proportional gain"; Kiic "Integral gain"; Kd "Derevative gain"
      mask TypeOptions P: Real power  | Reactive power
      mask DialogControl Container4 Prompt: General
      mask DialogControl Container5 Prompt: Current Controller
  mabc : Outport
  wires:
  Pref/1 -> Power Reference Controller/3(Pref)
  PLL & Measurements/1(VIbus) -> Power Reference Controller/1(VIbus)
  Power Reference Controller/1(m_abc) -> mabc/1
  Iabc/1 -> PLL & Measurements/2(I)
  Vabc/1 -> PLL & Measurements/1(V)
  Constant/1 -> Power Reference Controller/2(LVRT_iq)
  Qref/1 -> Power Reference Controller/4(Qref)

== system Solar_Plant_Harness/Solar Plant/Detailed/PV Plant & Controller/PV Plant/Converter/Average ==
  mabc : Inport
  Converter : ee_lib/Semiconductors & Converters/Converters/Average-Value Voltage Source Converter (Three-Phase)  port_option=ee.enum.threePhasePort.composite  frequency_option=ee.enum.converters.frequency.variable  input_option=ee.enum.converters.inputOption.ModWave  FRated=60 Hz  losses_parameterization=ee.enum.converters.losses.fixed  Pfixed=0.5 W  ks=0.01  kc1=1.7 V  kc2=0.01 Ohm  Ploss_vect=[100, 800, 1870, 3250, 4900] W  Irms_vect=[10, 100, 200, 300, 400] A  Vdc_nom=300 V  thermal_mass=30000 J/K  temperature_specify=off  temperature_priority=High  temperature=298.15 K  temperature_nominal_specify=off  temperature_nominal_value=1  temperature_nominal_unit=K
      settings: InternalSimscapePortConfiguration="{\"Bottom\":[],\"Left\":[{\"id\":\"ModWave\",\"label\":\"ModWave\",\"type\":\"input\"},{\"id\":\"N\",\"label\":\"~\",\"type\":\"foundation.electrical.three_phase\"}],\"Right\":[{\"id\":\"p\",\"label\":\"+\",\"type\":\"foundation.electrical.electrical\"},{\"id\":\"n\",\"label\":\"-\",\"type\":\"foundation.electrical.electrical\"}],\"Top\":[]}"
  Simulink-PS Converter : nesl_utility/Simulink-PS Converter  PhysicalDomain=network_engine_domain  SubClassName=ps_input  LeftPortType=input  RightPortType=output  PseudoPeriodic=off  Frequencies=[]  NoiseDistribution=none  NoiseParameters=[]  Unit=1  AffineConversion=off  FilteringAndDerivatives=provide  SimscapeFilterOrder=1  InputFilterTimeConstant=0.001  UdotUserProvided=0
  + : PMIOPort  Side=Left
  - : PMIOPort  Port=2  Side=Left
  ~ : PMIOPort  Port=3  Side=Right
  wires:
  mabc/1 -> Simulink-PS Converter/1
  connections:
  Simulink-PS Converter/RConn1 -- Converter/LConn1
  ~/RConn1 -- Converter/LConn2
  -/RConn1 -- Converter/RConn2
  +/RConn1 -- Converter/RConn1
